simulink model "cstr"  (R2019b)
settings: Solver=VariableStepAuto  StartTime=0.0  StopTime=500  RelTol=1e-3
model workspace (MATLAB code in the model file):
  | D = 52;
  | Ti = 90;
  | % Co = 0.8;
  | Cp = 0.844;
  | % Cino = 1;
  | H = -500;
  | % To = Ti + ((H*V)/(Q*Cp*D))*(2.4*10^15*exp(-2000/(To+459.67)));
  | % Co = (0.8*Q/V)/((Q/V)+(2.4*10^15*exp(-2000/(To+459.67))));)
  | Cao = 0;
  | To = 0;
values from neighbouring files (symbols this model uses):
  Q = 2.67    [code.m]
  V = 160.41    [code.m]
settings Model: Creator=sourabh  LastModifiedBy=sourabh

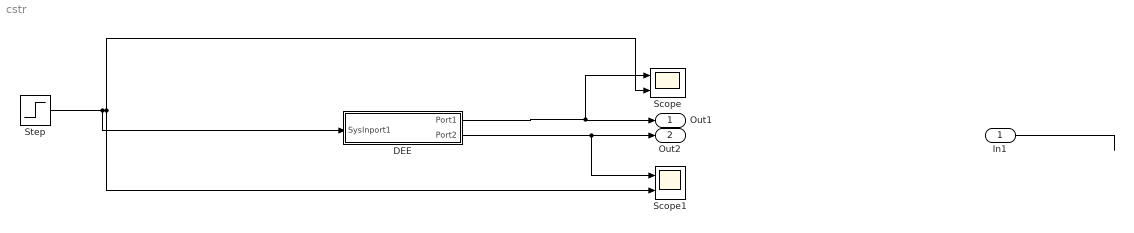
== system cstr ==
  In1 : Inport
  DEE : Subsystem  mask(Differential Equation Editor (DEE)){}
      settings: OpenFcn=diffeqed
      mask Display: disp('CSTR')
  Scope : Scope  NumInputPorts=2
  Scope1 : Scope  NumInputPorts=2
  Step : Step  Time=2  Before=0.8  After=0.8*1.1  SampleTime=1  VectorParams1D=off  ZeroCross=off
  Out1 : Outport
  Out2 : Outport  Port=2
  wires:
  In1/1 -> ?
  DEE/1(Port1) -> Out1/1, Scope/1
  DEE/2(Port2) -> Scope1/1, Out2/1
  Step/1 -> Scope1/2, Scope/2, DEE/1(SysInport1)

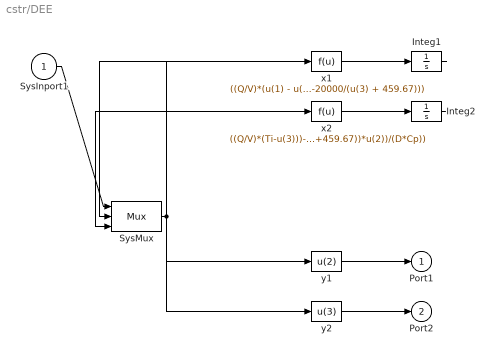
== system cstr/DEE ==
  SysInport1 : Inport
  Integ1 : Integrator  InitialCondition=0.0192
  Integ2 : Integrator  InitialCondition=98.8950
  SysMux : Mux  Inputs=3
  x1 : Fcn  Expr=((Q/V)*(u(1) - u(2))) - (u(2)*2.4*10^15*exp(-20000/(u(3) + 459.67)))
  x2 : Fcn  Expr=((Q/V)*(Ti-u(3)))-((H*2.4*10^15*exp(-20000/(u(3)+459.67))*u(2))/(D*Cp))
  y1 : Fcn  Expr=u(2)
  y2 : Fcn  Expr=u(3)
  Port1 : Outport
  Port2 : Outport  Port=2
  wires:
  SysInport1/1 -> SysMux/1
  SysMux/1 -> x1/1, x2/1, y1/1, y2/1
  x1/1 -> Integ1/1
  Integ1/1 -> SysMux/2
  x2/1 -> Integ2/1
  Integ2/1 -> SysMux/3
  y1/1 -> Port1/1
  y2/1 -> Port2/1
